simulink model "e"  (R2023a)
settings: Solver=VariableStepAuto  StartTime=0.0  StopTime=15  RelTol=1e-3
settings Model: Creator=eriknymobohne  LastModifiedBy=eriknymobohne

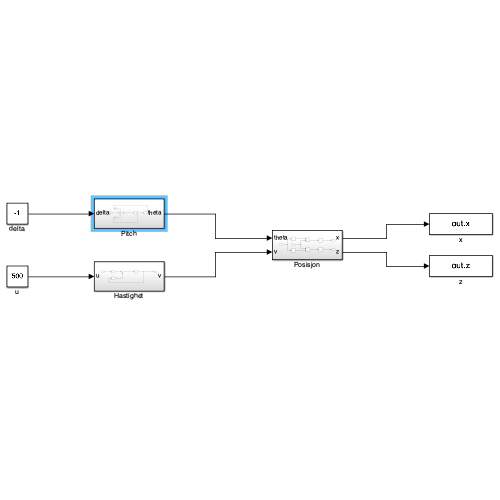
[thumbnail: Simulink's stored preview of the top-level diagram]
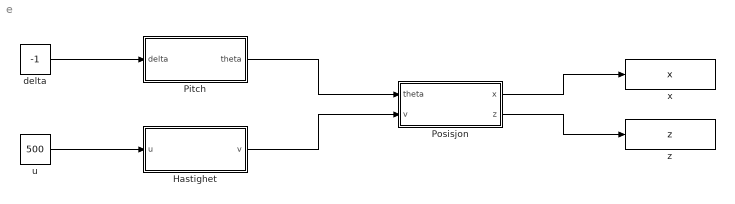
== system e ==
  Hastighet : Subsystem
  Pitch : Subsystem
  Posisjon : Subsystem
  delta : Constant  Value=-1
  u : Constant  Value=500
  x : ToWorkspace  VariableName=x  SaveFormat=Timeseries  SampleTime=-1
  z : ToWorkspace  VariableName=z  SaveFormat=Timeseries  SampleTime=-1
  wires:
  Pitch/1(theta) -> Posisjon/1(theta)
  u/1 -> Hastighet/1(u)
  Hastighet/1(v) -> Posisjon/2(v)
  Posisjon/2(z) -> z/1
  Posisjon/1(x) -> x/1
  delta/1 -> Pitch/1(delta)

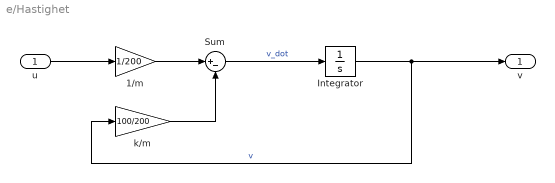
== system e/Hastighet ==
  u : Inport
  1/m : Gain  Gain=1/200
  Integrator : Integrator
  Sum : Sum  Inputs=|+-
  k/m : Gain  Gain=100/200
  v : Outport
  wires:
  Sum/1 -> Integrator/1  "v_dot"
  Integrator/1 -> k/m/1, v/1  "v"
  u/1 -> 1/m/1
  1/m/1 -> Sum/1
  k/m/1 -> Sum/2

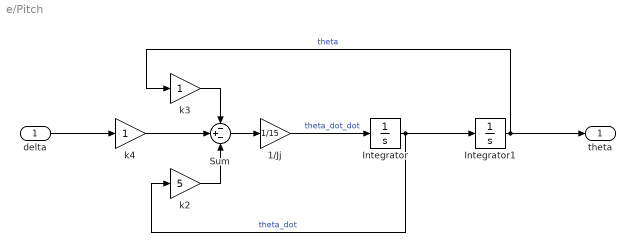
== system e/Pitch ==
  delta : Inport
  1/Jj : Gain  Gain=1/15
  Integrator : Integrator
  Integrator1 : Integrator
  Sum : Sum  Inputs=-+-
  k2 : Gain  Gain=5
  k3 : Gain
  k4 : Gain
  theta : Outport
  wires:
  delta/1 -> k4/1
  k4/1 -> Sum/2
  k2/1 -> Sum/3
  k3/1 -> Sum/1
  Sum/1 -> 1/Jj/1
  1/Jj/1 -> Integrator/1  "theta_dot_dot"
  Integrator/1 -> k2/1, Integrator1/1  "theta_dot"
  Integrator1/1 -> k3/1, theta/1  "theta"

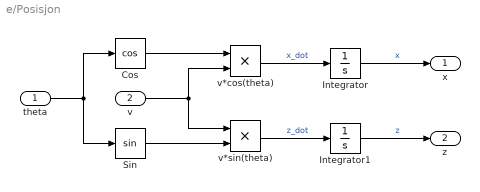
== system e/Posisjon ==
  theta : Inport
  v : Inport  Port=2
  Cos : Trigonometry  Operator=cos
  Integrator : Integrator
  Integrator1 : Integrator
  Sin : Trigonometry
  v*cos(theta) : Product
  v*sin(theta) : Product
  x : Outport
  z : Outport  Port=2
  wires:
  theta/1 -> Sin/1, Cos/1
  v/1 -> v*sin(theta)/1, v*cos(theta)/2
  Sin/1 -> v*sin(theta)/2
  Cos/1 -> v*cos(theta)/1
  v*cos(theta)/1 -> Integrator/1  "x_dot"
  Integrator/1 -> x/1  "x"
  v*sin(theta)/1 -> Integrator1/1  "z_dot"
  Integrator1/1 -> z/1  "z"
